simulink model "Logical_Ventilation"  (R2025b)
settings: Solver=VariableStepAuto  StartTime=0.0  StopTime=inf  RelTol=1e-3
PostLoadFcn:
  | load rel_humidity.mat;
  | load rel_humidity_heatedwire.mat;
  | load rel_humidityInput.mat;
libraries: slident x2, SignalEditorBlockLib x1
(part 1 of 3)
settings Model: DataDictionary=Logical_Ventilation_dict.sldd  Creator=ppatel  LastModifiedBy=ppatel
settings RTWCC: GPUComputeCapability=3.5

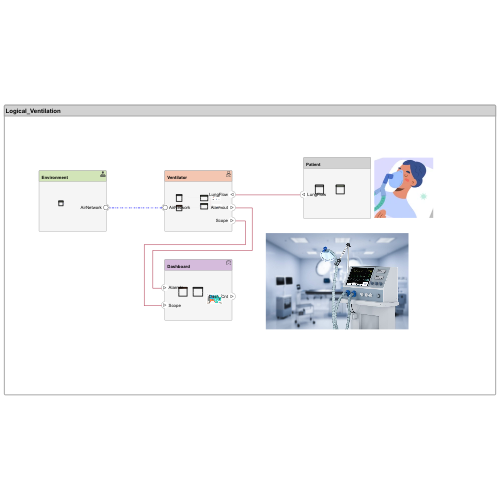
[thumbnail: Simulink's stored preview of the top-level diagram]
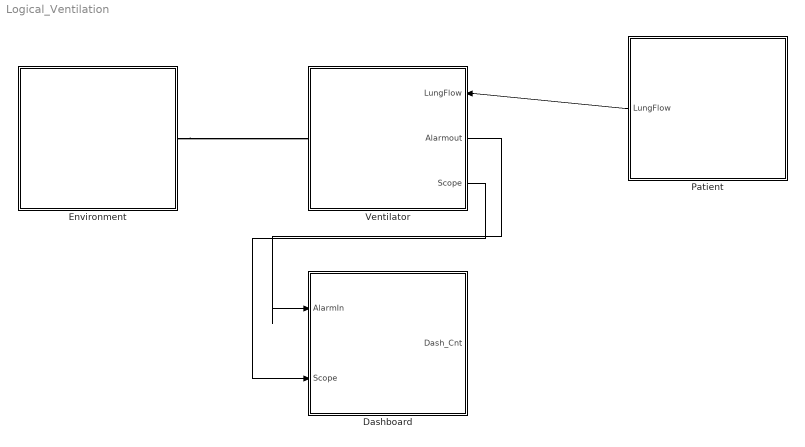
== system Logical_Ventilation ==
  Dashboard : Subsystem
      settings: PortSchema="{\"entries\":[{\"content\":{\"headerSize\":26,\"margin\":15,\"minimumSpacing\":25,\"sides\":[{\"content\":{\"connectorIds\":[\"In1\",\"In2\"]},\"type\":\"ConnectorPlacement.EquallySpacedRectSide\",\"uuid\":\"30d5a539-2c7a-40a6-b159-872080309fb0\"},{\"content\":{\"connectorIds\":[\"Out1\"],\"side\":\"RIGHT\"},\"type\":\"ConnectorPlacement.EquallySpacedRectSide\",\"uuid\":\"9c23b845-c6d3-461f-9717-3c81fce4740e\"},{\"content\":{\"side\":\"TOP\"},\"type\":\"ConnectorPlacement.EquallySpacedRectSide\",\"uuid\":\"23e2f61e-2083-47d3-9d3a-aca5cd4f1fc6\"}]},\"type\":\"ConnectorPlacement.EquallySpacedConnector\",\"uuid\":\"a2e9d942-417e-49d1-8834-66036fdf29fe\"}],\"packageUris\":[\"http://schema.mathworks.com/mf0/Connector/R2020b\"],\"version\":\"1.0\"}"
  Environment : Subsystem
      settings: PortSchema="{\"entries\":[{\"content\":{\"headerSize\":26,\"margin\":15,\"minimumSpacing\":25,\"sides\":[{\"content\":{},\"type\":\"ConnectorPlacement.EquallySpacedRectSide\",\"uuid\":\"30d5a539-2c7a-40a6-b159-872080309fb0\"},{\"content\":{\"connectorIds\":[\"RConn1\"],\"side\":\"RIGHT\"},\"type\":\"ConnectorPlacement.EquallySpacedRectSide\",\"uuid\":\"9c23b845-c6d3-461f-9717-3c81fce4740e\"},{\"content\":{\"side\":\"TOP\"},\"type\":\"ConnectorPlacement.EquallySpacedRectSide\",\"uuid\":\"23e2f61e-2083-47d3-9d3a-aca5cd4f1fc6\"}]},\"type\":\"ConnectorPlacement.EquallySpacedConnector\",\"uuid\":\"a2e9d942-417e-49d1-8834-66036fdf29fe\"}],\"packageUris\":[\"http://schema.mathworks.com/mf0/Connector/R2020b\"],\"version\":\"1.0\"}"
  Patient : Subsystem
      settings: PortSchema="{\"entries\":[{\"content\":{\"headerSize\":26,\"margin\":15,\"minimumSpacing\":25,\"sides\":[{\"content\":{\"connectorIds\":[\"Out1\"]},\"type\":\"ConnectorPlacement.EquallySpacedRectSide\",\"uuid\":\"30d5a539-2c7a-40a6-b159-872080309fb0\"},{\"content\":{\"side\":\"RIGHT\"},\"type\":\"ConnectorPlacement.EquallySpacedRectSide\",\"uuid\":\"9c23b845-c6d3-461f-9717-3c81fce4740e\"},{\"content\":{\"side\":\"TOP\"},\"type\":\"ConnectorPlacement.EquallySpacedRectSide\",\"uuid\":\"23e2f61e-2083-47d3-9d3a-aca5cd4f1fc6\"}]},\"type\":\"ConnectorPlacement.EquallySpacedConnector\",\"uuid\":\"a2e9d942-417e-49d1-8834-66036fdf29fe\"}],\"packageUris\":[\"http://schema.mathworks.com/mf0/Connector/R2020b\"],\"version\":\"1.0\"}"
  Ventilator : Subsystem
      settings: PortSchema="{\"entries\":[{\"content\":{\"headerSize\":26,\"margin\":15,\"minimumSpacing\":25,\"sides\":[{\"content\":{\"connectorIds\":[\"RConn1\"]},\"type\":\"ConnectorPlacement.EquallySpacedRectSide\",\"uuid\":\"30d5a539-2c7a-40a6-b159-872080309fb0\"},{\"content\":{\"connectorIds\":[\"In1\",\"Out1\",\"Out2\"],\"side\":\"RIGHT\"},\"type\":\"ConnectorPlacement.EquallySpacedRectSide\",\"uuid\":\"9c23b845-c6d3-461f-9717-3c81fce4740e\"},{\"content\":{\"side\":\"TOP\"},\"type\":\"ConnectorPlacement.EquallySpacedRectSide\",\"uuid\":\"23e2f61e-2083-47d3-9d3a-aca5cd4f1fc6\"}]},\"type\":\"ConnectorPlacement.EquallySpacedConnector\",\"uuid\":\"a2e9d942-417e-49d1-8834-66036fdf29fe\"}],\"packageUris\":[\"http://schema.mathworks.com/mf0/Connector/R2020b\"],\"version\":\"1.0\"}"
  wires:
  Patient/1(LungFlow) -> Ventilator/1(LungFlow)
  Ventilator/1(Alarmout) -> Dashboard/1(AlarmIn)
  Ventilator/2(Scope) -> Dashboard/2(Scope)
  connections:
  Environment/RConn1 -- Ventilator/RConn1

== system Logical_Ventilation/Dashboard ==
  Bus Element In1 : Inport  OutputPortMessageModes=m  PortName=AlarmIn
  Bus Element In2 : Inport  Port=2  PortName=Scope
  Alarm : Subsystem
      settings: PortSchema="{\"entries\":[{\"content\":{\"headerSize\":26,\"margin\":15,\"minimumSpacing\":25,\"sides\":[{\"content\":{\"connectorIds\":[\"In1\"]},\"type\":\"ConnectorPlacement.EquallySpacedRectSide\",\"uuid\":\"30d5a539-2c7a-40a6-b159-872080309fb0\"},{\"content\":{\"side\":\"RIGHT\"},\"type\":\"ConnectorPlacement.EquallySpacedRectSide\",\"uuid\":\"9c23b845-c6d3-461f-9717-3c81fce4740e\"},{\"content\":{\"side\":\"TOP\"},\"type\":\"ConnectorPlacement.EquallySpacedRectSide\",\"uuid\":\"23e2f61e-2083-47d3-9d3a-aca5cd4f1fc6\"}]},\"type\":\"ConnectorPlacement.EquallySpacedConnector\",\"uuid\":\"a2e9d942-417e-49d1-8834-66036fdf29fe\"}],\"packageUris\":[\"http://schema.mathworks.com/mf0/Connector/R2020b\"],\"version\":\"1.0\"}"
  Controls & Display : Subsystem
      settings: PortSchema="{\"entries\":[{\"content\":{\"headerSize\":26,\"margin\":15,\"minimumSpacing\":25,\"sides\":[{\"content\":{\"connectorIds\":[\"In1\"]},\"type\":\"ConnectorPlacement.EquallySpacedRectSide\",\"uuid\":\"30d5a539-2c7a-40a6-b159-872080309fb0\"},{\"content\":{\"connectorIds\":[\"Out1\"],\"side\":\"RIGHT\"},\"type\":\"ConnectorPlacement.EquallySpacedRectSide\",\"uuid\":\"9c23b845-c6d3-461f-9717-3c81fce4740e\"},{\"content\":{\"side\":\"TOP\"},\"type\":\"ConnectorPlacement.EquallySpacedRectSide\",\"uuid\":\"23e2f61e-2083-47d3-9d3a-aca5cd4f1fc6\"}]},\"type\":\"ConnectorPlacement.EquallySpacedConnector\",\"uuid\":\"a2e9d942-417e-49d1-8834-66036fdf29fe\"}],\"packageUris\":[\"http://schema.mathworks.com/mf0/Connector/R2020b\"],\"version\":\"1.0\"}"
  Bus Element Out1 : Outport  PortName=Dash_Cnt
  wires:
  Controls & Display/1(Dash_Cnt) -> Bus Element Out1/1
  Bus Element In1/1 -> Alarm/1(AlarmIn)

== system Logical_Ventilation/Environment ==
  Source_Sink_Air : Subsystem
      settings: PortSchema="{\"entries\":[{\"content\":{\"headerSize\":26,\"margin\":15,\"minimumSpacing\":25,\"sides\":[{\"content\":{},\"type\":\"ConnectorPlacement.EquallySpacedRectSide\",\"uuid\":\"30d5a539-2c7a-40a6-b159-872080309fb0\"},{\"content\":{\"connectorIds\":[\"RConn1\"],\"side\":\"RIGHT\"},\"type\":\"ConnectorPlacement.EquallySpacedRectSide\",\"uuid\":\"9c23b845-c6d3-461f-9717-3c81fce4740e\"},{\"content\":{\"side\":\"TOP\"},\"type\":\"ConnectorPlacement.EquallySpacedRectSide\",\"uuid\":\"23e2f61e-2083-47d3-9d3a-aca5cd4f1fc6\"}]},\"type\":\"ConnectorPlacement.EquallySpacedConnector\",\"uuid\":\"a2e9d942-417e-49d1-8834-66036fdf29fe\"}],\"packageUris\":[\"http://schema.mathworks.com/mf0/Connector/R2020b\"],\"version\":\"1.0\"}"
  AirNetwork : PMIOPort  Side=Right  ConnectionType=Bus: AirSupply
  connections:
  Source_Sink_Air/RConn1 -- AirNetwork/RConn1

== system Logical_Ventilation/Patient ==
  Lung : Subsystem
      settings: PortSchema="{\"entries\":[{\"content\":{\"headerSize\":26,\"margin\":15,\"minimumSpacing\":25,\"sides\":[{\"content\":{},\"type\":\"ConnectorPlacement.EquallySpacedRectSide\",\"uuid\":\"30d5a539-2c7a-40a6-b159-872080309fb0\"},{\"content\":{\"side\":\"RIGHT\"},\"type\":\"ConnectorPlacement.EquallySpacedRectSide\",\"uuid\":\"9c23b845-c6d3-461f-9717-3c81fce4740e\"},{\"content\":{\"side\":\"TOP\"},\"type\":\"ConnectorPlacement.EquallySpacedRectSide\",\"uuid\":\"23e2f61e-2083-47d3-9d3a-aca5cd4f1fc6\"}]},\"type\":\"ConnectorPlacement.EquallySpacedConnector\",\"uuid\":\"a2e9d942-417e-49d1-8834-66036fdf29fe\"}],\"packageUris\":[\"http://schema.mathworks.com/mf0/Connector/R2020b\"],\"version\":\"1.0\"}"
  Mask : Subsystem
      settings: PortSchema="{\"entries\":[{\"content\":{\"headerSize\":26,\"margin\":15,\"minimumSpacing\":25,\"sides\":[{\"content\":{},\"type\":\"ConnectorPlacement.EquallySpacedRectSide\",\"uuid\":\"30d5a539-2c7a-40a6-b159-872080309fb0\"},{\"content\":{\"side\":\"RIGHT\"},\"type\":\"ConnectorPlacement.EquallySpacedRectSide\",\"uuid\":\"9c23b845-c6d3-461f-9717-3c81fce4740e\"},{\"content\":{\"side\":\"TOP\"},\"type\":\"ConnectorPlacement.EquallySpacedRectSide\",\"uuid\":\"23e2f61e-2083-47d3-9d3a-aca5cd4f1fc6\"}]},\"type\":\"ConnectorPlacement.EquallySpacedConnector\",\"uuid\":\"a2e9d942-417e-49d1-8834-66036fdf29fe\"}],\"packageUris\":[\"http://schema.mathworks.com/mf0/Connector/R2020b\"],\"version\":\"1.0\"}"
  Bus Element Out1 : Outport  PortName=LungFlow

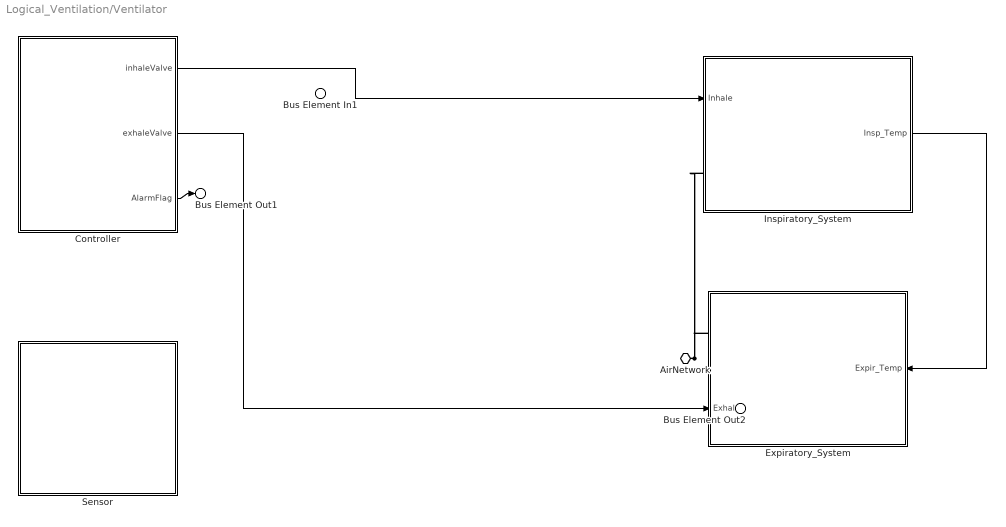
== system Logical_Ventilation/Ventilator ==
  Bus Element In1 : Inport  PortName=LungFlow
  Controller : Subsystem
      settings: PortSchema="{\"entries\":[{\"content\":{\"headerSize\":26,\"margin\":15,\"minimumSpacing\":25,\"sides\":[{\"content\":{},\"type\":\"ConnectorPlacement.EquallySpacedRectSide\",\"uuid\":\"a6b9ac84-da55-41fa-8d69-203bfd5ed961\"},{\"content\":{\"connectorIds\":[\"Out1\",\"Out2\",\"Out3\"],\"side\":\"RIGHT\"},\"type\":\"ConnectorPlacement.EquallySpacedRectSide\",\"uuid\":\"59cae5fa-9dfc-477f-ab42-7807dc2f7843\"},{\"content\":{\"side\":\"TOP\"},\"type\":\"ConnectorPlacement.EquallySpacedRectSide\",\"uuid\":\"b518b906-755c-4724-95bc-822fd83ee92e\"}]},\"type\":\"ConnectorPlacement.EquallySpacedConnector\",\"uuid\":\"935b65cc-f99b-4334-a861-ce966d6a0f10\"}],\"packageUris\":[\"http://schema.mathworks.com/mf0/Connector/R2020b\"],\"version\":\"1.0\"}"
  Expiratory_System : Subsystem
      settings: PortSchema="{\"entries\":[{\"content\":{\"headerSize\":26,\"margin\":15,\"minimumSpacing\":25,\"sides\":[{\"content\":{\"connectorIds\":[\"LConn1\",\"In1\"]},\"type\":\"ConnectorPlacement.EquallySpacedRectSide\",\"uuid\":\"30d5a539-2c7a-40a6-b159-872080309fb0\"},{\"content\":{\"connectorIds\":[\"In2\"],\"side\":\"RIGHT\"},\"type\":\"ConnectorPlacement.EquallySpacedRectSide\",\"uuid\":\"9c23b845-c6d3-461f-9717-3c81fce4740e\"},{\"content\":{\"side\":\"TOP\"},\"type\":\"ConnectorPlacement.EquallySpacedRectSide\",\"uuid\":\"23e2f61e-2083-47d3-9d3a-aca5cd4f1fc6\"}]},\"type\":\"ConnectorPlacement.EquallySpacedConnector\",\"uuid\":\"a2e9d942-417e-49d1-8834-66036fdf29fe\"}],\"packageUris\":[\"http://schema.mathworks.com/mf0/Connector/R2020b\"],\"version\":\"1.0\"}"
  Inspiratory_System : Subsystem
      settings: PortSchema="{\"entries\":[{\"content\":{\"headerSize\":26,\"margin\":15,\"minimumSpacing\":25,\"sides\":[{\"content\":{\"connectorIds\":[\"In1\",\"LConn1\"]},\"type\":\"ConnectorPlacement.EquallySpacedRectSide\",\"uuid\":\"30d5a539-2c7a-40a6-b159-872080309fb0\"},{\"content\":{\"connectorIds\":[\"Out1\"],\"side\":\"RIGHT\"},\"type\":\"ConnectorPlacement.EquallySpacedRectSide\",\"uuid\":\"9c23b845-c6d3-461f-9717-3c81fce4740e\"},{\"content\":{\"side\":\"TOP\"},\"type\":\"ConnectorPlacement.EquallySpacedRectSide\",\"uuid\":\"23e2f61e-2083-47d3-9d3a-aca5cd4f1fc6\"}]},\"type\":\"ConnectorPlacement.EquallySpacedConnector\",\"uuid\":\"a2e9d942-417e-49d1-8834-66036fdf29fe\"}],\"packageUris\":[\"http://schema.mathworks.com/mf0/Connector/R2020b\"],\"version\":\"1.0\"}"
  Sensor : Subsystem
      settings: PortSchema="{\"entries\":[{\"content\":{\"headerSize\":26,\"margin\":15,\"minimumSpacing\":25,\"sides\":[{\"content\":{},\"type\":\"ConnectorPlacement.EquallySpacedRectSide\",\"uuid\":\"30d5a539-2c7a-40a6-b159-872080309fb0\"},{\"content\":{\"side\":\"RIGHT\"},\"type\":\"ConnectorPlacement.EquallySpacedRectSide\",\"uuid\":\"9c23b845-c6d3-461f-9717-3c81fce4740e\"},{\"content\":{\"side\":\"TOP\"},\"type\":\"ConnectorPlacement.EquallySpacedRectSide\",\"uuid\":\"23e2f61e-2083-47d3-9d3a-aca5cd4f1fc6\"}]},\"type\":\"ConnectorPlacement.EquallySpacedConnector\",\"uuid\":\"a2e9d942-417e-49d1-8834-66036fdf29fe\"}],\"packageUris\":[\"http://schema.mathworks.com/mf0/Connector/R2020b\"],\"version\":\"1.0\"}"
  AirNetwork : PMIOPort  Side=Right  ConnectionType=Bus: AirSupply
  Bus Element Out1 : Outport  PortName=Alarmout
  Bus Element Out2 : Outport  Port=2  PortName=Scope
  wires:
  Inspiratory_System/1(Insp_Temp) -> Expiratory_System/2(Expir_Temp)
  Controller/1(inhaleValve) -> Inspiratory_System/1(Inhale)
  Controller/2(exhaleValve) -> Expiratory_System/1(Exhale)
  Controller/3(AlarmFlag) -> Bus Element Out1/1
  connections:
  Inspiratory_System/LConn1 -- Expiratory_System/LConn1 -- AirNetwork/RConn1

== system Logical_Ventilation/Dashboard/Alarm ==
  AlarmIn : Inport  OutDataTypeStr=Bus: Alarm
  Control_Failure : LampBlock  LabelPosition=Hide  DefaultColor=[192.0, 192.0, 192.0]
  High_Insp_Pressure : LampBlock  LabelPosition=Hide  DefaultColor=[192.0, 192.0, 192.0]
  Message Receive : Receive  InputPortMessageModes=m
  Terminator : Terminator
  wires:
  AlarmIn/1 -> Message Receive/1
  Message Receive/1 -> Terminator/1

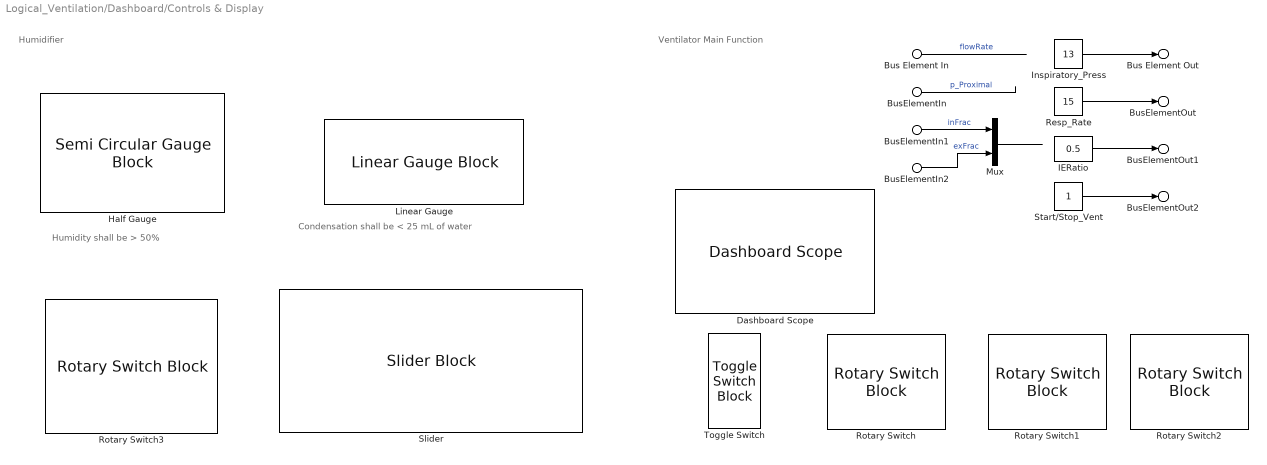
== system Logical_Ventilation/Dashboard/Controls & Display ==
  note: Condensation shall be < 25 mL of water
  note: Humidity shall be > 50%
  note: Humidifier
  note: Ventilator Main Function
  Bus Element In : Inport  PortName=Scope  Element=flowRate
  BusElementIn : Inport  PortName=Scope  Element=pProximal
  BusElementIn1 : Inport  PortName=Scope  Element=inValveFrac
  BusElementIn2 : Inport  PortName=Scope  Element=exValve
  Dashboard Scope : DashboardScope  FontColor=[0.0, 0.0, 0.0]
  Half Gauge : SemiCircularGaugeBlock  FontColor=[0.0, 0.0, 0.0]
  IERatio : Constant  Value=0.5
  Inspiratory_Press : Constant  Value=13  OutDataTypeStr=uint8
  Linear Gauge : LinearGaugeBlock  ScaleMax=50  FontColor=[0.0, 0.0, 0.0]
  Mux : Mux  Inputs=2
  Resp_Rate : Constant  Value=15  OutDataTypeStr=uint8
  Rotary Switch{,1..3} (4 alike) : RotarySwitchBlock
  Slider : SliderBlock  ScaleMax=50  TickInterval=5
  Start/Stop_Vent : Constant  OutDataTypeStr=boolean
  Toggle Switch : ToggleSwitchBlock
  Bus Element Out : Outport  PortName=Dash_Cnt  Element=insp_press
  BusElementOut : Outport  PortName=Dash_Cnt  Element=RR
  BusElementOut1 : Outport  PortName=Dash_Cnt  Element=IERatio
  BusElementOut2 : Outport  PortName=Dash_Cnt  Element=StartStopVent
  wires:
  Resp_Rate/1 -> BusElementOut/1
  IERatio/1 -> BusElementOut1/1
  Inspiratory_Press/1 -> Bus Element Out/1
  Start/Stop_Vent/1 -> BusElementOut2/1
  Bus Element In/1 -> ?  "flowRate"
  BusElementIn/1 -> ?  "p_Proximal"
  Mux/1 -> ?
  BusElementIn2/1 -> Mux/2  "exFrac"
  BusElementIn1/1 -> Mux/1  "inFrac"

== system Logical_Ventilation/Environment/Source_Sink_Air ==
  AirNetwork : PMIOPort  Side=Right

== system Logical_Ventilation/Patient/Lung ==

== system Logical_Ventilation/Patient/Mask ==

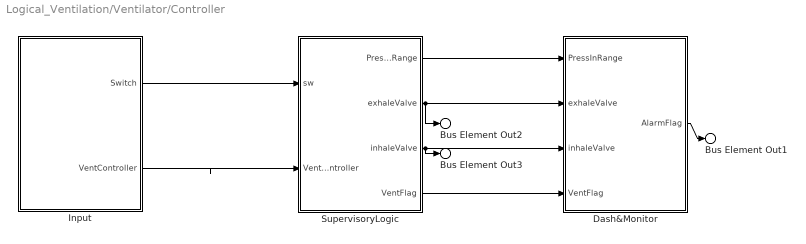
== system Logical_Ventilation/Ventilator/Controller ==
  Dash&Monitor : Subsystem
      settings: PortSchema="{\"entries\":[{\"content\":{\"headerSize\":26,\"margin\":15,\"minimumSpacing\":25,\"sides\":[{\"content\":{\"connectorIds\":[\"In1\",\"In3\",\"In2\",\"In4\"]},\"type\":\"ConnectorPlacement.EquallySpacedRectSide\",\"uuid\":\"a6b9ac84-da55-41fa-8d69-203bfd5ed961\"},{\"content\":{\"connectorIds\":[\"Out1\"],\"side\":\"RIGHT\"},\"type\":\"ConnectorPlacement.EquallySpacedRectSide\",\"uuid\":\"59cae5fa-9dfc-477f-ab42-7807dc2f7843\"},{\"content\":{\"side\":\"TOP\"},\"type\":\"ConnectorPlacement.EquallySpacedRectSide\",\"uuid\":\"b518b906-755c-4724-95bc-822fd83ee92e\"}]},\"type\":\"ConnectorPlacement.EquallySpacedConnector\",\"uuid\":\"935b65cc-f99b-4334-a861-ce966d6a0f10\"}],\"packageUris\":[\"http://schema.mathworks.com/mf0/Connector/R2020b\"],\"version\":\"1.0\"}"
  Input : Subsystem
      settings: PortSchema="{\"entries\":[{\"content\":{\"headerSize\":26,\"margin\":15,\"minimumSpacing\":25,\"sides\":[{\"content\":{},\"type\":\"ConnectorPlacement.EquallySpacedRectSide\",\"uuid\":\"a6b9ac84-da55-41fa-8d69-203bfd5ed961\"},{\"content\":{\"connectorIds\":[\"Out1\",\"Out2\"],\"side\":\"RIGHT\"},\"type\":\"ConnectorPlacement.EquallySpacedRectSide\",\"uuid\":\"59cae5fa-9dfc-477f-ab42-7807dc2f7843\"},{\"content\":{\"side\":\"TOP\"},\"type\":\"ConnectorPlacement.EquallySpacedRectSide\",\"uuid\":\"b518b906-755c-4724-95bc-822fd83ee92e\"}]},\"type\":\"ConnectorPlacement.EquallySpacedConnector\",\"uuid\":\"935b65cc-f99b-4334-a861-ce966d6a0f10\"}],\"packageUris\":[\"http://schema.mathworks.com/mf0/Connector/R2020b\"],\"version\":\"1.0\"}"
  SupervisoryLogic : Stateflow chart  TreatAsAtomicUnit=on
      settings: PortSchema="{\"entries\":[{\"content\":{\"headerSize\":26,\"margin\":15,\"minimumSpacing\":25,\"sides\":[{\"content\":{\"connectorIds\":[\"In1\",\"In2\"]},\"type\":\"ConnectorPlacement.EquallySpacedRectSide\",\"uuid\":\"a6b9ac84-da55-41fa-8d69-203bfd5ed961\"},{\"content\":{\"connectorIds\":[\"Out1\",\"Out2\",\"Out3\",\"Out4\"],\"side\":\"RIGHT\"},\"type\":\"ConnectorPlacement.EquallySpacedRectSide\",\"uuid\":\"59cae5fa-9dfc-477f-ab42-7807dc2f7843\"},{\"content\":{\"side\":\"TOP\"},\"type\":\"ConnectorPlacement.EquallySpacedRectSide\",\"uuid\":\"b518b906-755c-4724-95bc-822fd83ee92e\"}]},\"type\":\"ConnectorPlacement.EquallySpacedConnector\",\"uuid\":\"935b65cc-f99b-4334-a861-ce966d6a0f10\"}],\"packageUris\":[\"http://schema.mathworks.com/mf0/Connector/R2020b\"],\"version\":\"1.0\"}"
  Bus Element Out3 : Outport  PortName=inhaleValve
  Bus Element Out2 : Outport  Port=2  PortName=exhaleValve
  Bus Element Out1 : Outport  InputPortMessageModes=m  Port=3  PortName=AlarmFlag
  wires:
  Input/2(VentController) -> SupervisoryLogic/2(VentController)
  Input/1(Switch) -> SupervisoryLogic/1(sw)
  SupervisoryLogic/1(PressInRange) -> Dash&Monitor/1(PressInRange)
  Dash&Monitor/1(AlarmFlag) -> Bus Element Out1/1
  SupervisoryLogic/2(exhaleValve) -> Dash&Monitor/3(exhaleValve), Bus Element Out2/1
  SupervisoryLogic/3(inhaleValve) -> Dash&Monitor/2(inhaleValve), Bus Element Out3/1
  SupervisoryLogic/4(VentFlag) -> Dash&Monitor/4(VentFlag)

== system Logical_Ventilation/Ventilator/Expiratory_System ==
  Bus Element In2 : Inport  PortName=Exhale
  Bus Element In1 : Inport  Port=2  PortName=Expir_Temp
  Expiratory_Tube : Subsystem
      settings: PortSchema="{\"entries\":[{\"content\":{\"headerSize\":26,\"margin\":15,\"minimumSpacing\":25,\"sides\":[{\"content\":{},\"type\":\"ConnectorPlacement.EquallySpacedRectSide\",\"uuid\":\"30d5a539-2c7a-40a6-b159-872080309fb0\"},{\"content\":{\"connectorIds\":[\"In1\"],\"side\":\"RIGHT\"},\"type\":\"ConnectorPlacement.EquallySpacedRectSide\",\"uuid\":\"9c23b845-c6d3-461f-9717-3c81fce4740e\"},{\"content\":{\"side\":\"TOP\"},\"type\":\"ConnectorPlacement.EquallySpacedRectSide\",\"uuid\":\"23e2f61e-2083-47d3-9d3a-aca5cd4f1fc6\"}]},\"type\":\"ConnectorPlacement.EquallySpacedConnector\",\"uuid\":\"a2e9d942-417e-49d1-8834-66036fdf29fe\"}],\"packageUris\":[\"http://schema.mathworks.com/mf0/Connector/R2020b\"],\"version\":\"1.0\"}"
  CO2Delivery : PMIOPort  Side=Left
  wires:
  Bus Element In1/1 -> Expiratory_Tube/1(ExpirTube_Temp)

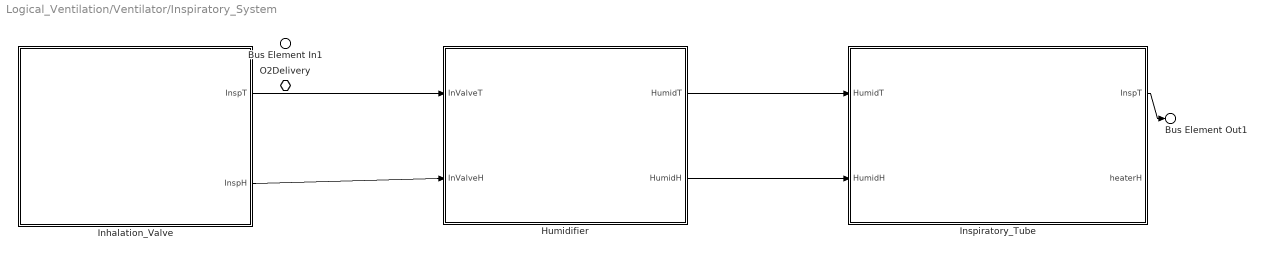
== system Logical_Ventilation/Ventilator/Inspiratory_System ==
  Bus Element In1 : Inport  PortName=Inhale
  Humidifier : Subsystem
      settings: PortSchema="{\"entries\":[{\"content\":{\"headerSize\":26,\"margin\":15,\"minimumSpacing\":25,\"sides\":[{\"content\":{\"connectorIds\":[\"In1\",\"In2\"]},\"type\":\"ConnectorPlacement.EquallySpacedRectSide\",\"uuid\":\"ac1af519-5858-4e19-8afa-0bef01d30598\"},{\"content\":{\"connectorIds\":[\"Out1\",\"Out2\"],\"side\":\"RIGHT\"},\"type\":\"ConnectorPlacement.EquallySpacedRectSide\",\"uuid\":\"9f8fa7b0-aa05-445f-8c6b-48bc3d0cae28\"},{\"content\":{\"side\":\"TOP\"},\"type\":\"ConnectorPlacement.EquallySpacedRectSide\",\"uuid\":\"07b6012d-ab32-4246-afe0-d86d9feed365\"}]},\"type\":\"ConnectorPlacement.EquallySpacedConnector\",\"uuid\":\"49d8837b-4b9b-40fe-b41d-d869734f4da7\"}],\"packageUris\":[\"http://schema.mathworks.com/mf0/Connector/R2020b\"],\"version\":\"1.0\"}"
  Inhalation_Valve : Subsystem
      settings: PortSchema="{\"entries\":[{\"content\":{\"headerSize\":26,\"margin\":15,\"minimumSpacing\":25,\"sides\":[{\"content\":{},\"type\":\"ConnectorPlacement.EquallySpacedRectSide\",\"uuid\":\"30d5a539-2c7a-40a6-b159-872080309fb0\"},{\"content\":{\"connectorIds\":[\"Out1\",\"Out2\"],\"side\":\"RIGHT\"},\"type\":\"ConnectorPlacement.EquallySpacedRectSide\",\"uuid\":\"9c23b845-c6d3-461f-9717-3c81fce4740e\"},{\"content\":{\"side\":\"TOP\"},\"type\":\"ConnectorPlacement.EquallySpacedRectSide\",\"uuid\":\"23e2f61e-2083-47d3-9d3a-aca5cd4f1fc6\"}]},\"type\":\"ConnectorPlacement.EquallySpacedConnector\",\"uuid\":\"a2e9d942-417e-49d1-8834-66036fdf29fe\"}],\"packageUris\":[\"http://schema.mathworks.com/mf0/Connector/R2020b\"],\"version\":\"1.0\"}"
  Inspiratory_Tube : Subsystem
      settings: PortSchema="{\"entries\":[{\"content\":{\"headerSize\":26,\"margin\":15,\"minimumSpacing\":25,\"sides\":[{\"content\":{\"connectorIds\":[\"In2\",\"In1\"]},\"type\":\"ConnectorPlacement.EquallySpacedRectSide\",\"uuid\":\"30d5a539-2c7a-40a6-b159-872080309fb0\"},{\"content\":{\"connectorIds\":[\"Out1\",\"Out2\"],\"side\":\"RIGHT\"},\"type\":\"ConnectorPlacement.EquallySpacedRectSide\",\"uuid\":\"9c23b845-c6d3-461f-9717-3c81fce4740e\"},{\"content\":{\"side\":\"TOP\"},\"type\":\"ConnectorPlacement.EquallySpacedRectSide\",\"uuid\":\"23e2f61e-2083-47d3-9d3a-aca5cd4f1fc6\"}]},\"type\":\"ConnectorPlacement.EquallySpacedConnector\",\"uuid\":\"a2e9d942-417e-49d1-8834-66036fdf29fe\"}],\"packageUris\":[\"http://schema.mathworks.com/mf0/Connector/R2020b\"],\"version\":\"1.0\"}"
  O2Delivery : PMIOPort  Side=Left
  Bus Element Out1 : Outport  PortName=Insp_Temp
  wires:
  Inspiratory_Tube/1(InspT) -> Bus Element Out1/1
  Humidifier/2(HumidH) -> Inspiratory_Tube/1(HumidH)
  Humidifier/1(HumidT) -> Inspiratory_Tube/2(HumidT)
  Inhalation_Valve/1(InspT) -> Humidifier/1(InValveT)
  Inhalation_Valve/2(InspH) -> Humidifier/2(InValveH)

== system Logical_Ventilation/Ventilator/Sensor ==
